simulink model "mpc_simulation_regulation"  (R2022a)
settings: Solver=VariableStepAuto  StartTime=0.0  StopTime=10  RelTol=1e-3
InitFcn:
  | mpc_example_regulation
values from neighbouring files (symbols this model uses):
  absolute_encoder_counts_per_revolution = 128    [ELEN90064_Project_Parameters.m]
  C = [0 1 0 0 0]    [DesignProjectP2.m]    (also in DesignProjectP3.m = [1 0 0 0 0; DesignProject_OffsetP3.m = [1 0 0 0 0; mpc_example_regulation.m = [1 0 0 0 0; mpc_example_tracking.m = [1 0 0 0 0)
  Dp = c2d(Gp, T, 'zoh')    [DesignProject_OffsetP3.m]    (also in mpc_example_regulation.m; mpc_example_tracking.m)
  gyro_sigma_drift = deg2rad(5)    [ELEN90064_Project_Parameters.m]
  init = [theta_m_init; theta_l_init; thetadot_m_init; thetadot_l_init; Ia_init]    [ELEN90064_Project_Parameters.m]
  L_disc = L_disct'    [DesignProject_OffsetP3.m]    (also in mpc_example_regulation.m; mpc_example_tracking.m)
libraries: mpclib x1
settings Model: Creator=pbeuchat  LastModifiedBy=Admin
settings SolverCC: AlgebraicLoopSolver=TrustRegion
settings DebuggingCC: UnconnectedInputMsg=warning  UnconnectedOutputMsg=warning  UnconnectedLineMsg=warning  SFMachineParentedDataDiag=warning
settings RTWCC: DLArmComputeVersion=19.05

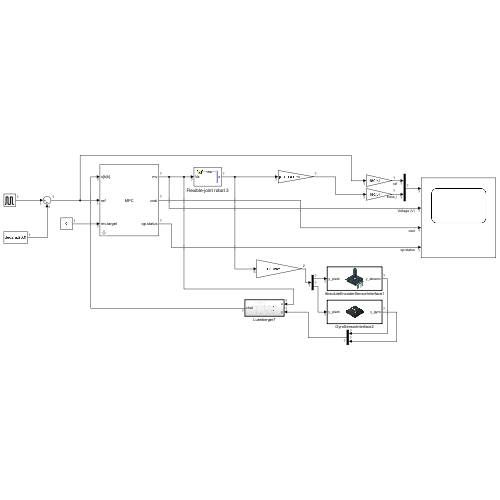
[thumbnail: Simulink's stored preview of the top-level diagram]
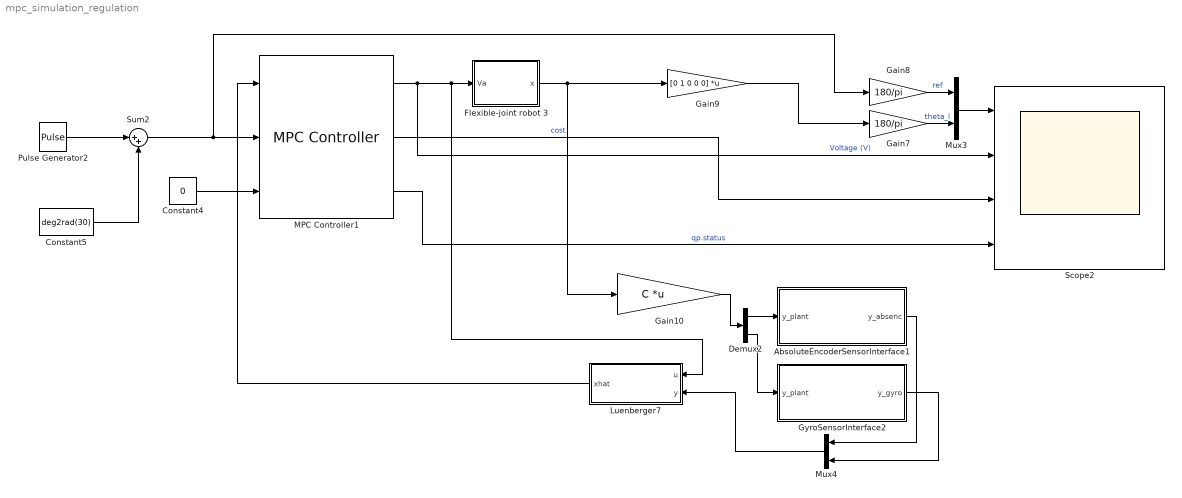
== system mpc_simulation_regulation ==
  AbsoluteEncoderSensorInterface1 : Subsystem  TreatAsAtomicUnit=on
      mask Display: image('$imagefile'); % Use "Edit Image" on toolstrip to change.
  Constant4 : Constant  Value=0
  Constant5 : Constant  Value=deg2rad(30)
  Demux2 : Demux  Outputs=2
  Flexible-joint robot 3 : Subsystem
      mask Display: image('$imagefile'); % Use "Edit Image" on toolstrip to change.
  Gain10 : Gain  Gain=C  Multiplication=Matrix(K*u) (u vector)
  Gain7 : Gain  Gain=180/pi
  Gain8 : Gain  Gain=180/pi
  Gain9 : Gain  Gain=[0 1 0 0 0]  Multiplication=Matrix(K*u)
  GyroSensorInterface2 : Subsystem  TreatAsAtomicUnit=on
      mask Display: image('$imagefile'); % Use "Edit Image" on toolstrip to change.
  Luenberger7 : Subsystem  TreatAsAtomicUnit=on
  MPC Controller1 : mpclib/MPC Controller  SCDEnableBlockLinearizationSpecification=on  mpcobj=mpc_obj  x0=mpc_initial_state  is_multiple=0  enable_value=0  return_u0=off  updateMPCinCallerWorkspace=on  md_inport=off  mv_inport=off  uref_inport=on  return_cost=on  return_mvseq=off  return_qpstatus=on  return_xseq=off  return_state=off  return_ovseq=off  state_inport=on  umin_inport=off  umax_inport=off  ymin_inport=off  ymax_inport=off  cc_inport=off  ywt_inport=off  uwt_inport=off  duwt_inport=off  rhoeps_inport=off  pm_inport=off  MaximumP=10  HorizonChoice=FixedHorizon  n_ts=0.02  n_p=20  n_mv=1  n_md=0  n_ud=0  n_mo=13  n_uo=0  BlockDataType=double  SampleTimeInherited=off  switch_inport=off
  Mux3 : Mux  Inputs=2
  Mux4 : Mux  Inputs=2
  Pulse Generator2 : DiscretePulseGenerator  PulseType=Time based  Amplitude=deg2rad(30)  Period=5  PulseWidth=50
  Scope2 : Scope  NumInputPorts=4
  Sum2 : Sum  Inputs=|++
  wires:
  Gain10/1 -> Demux2/1
  AbsoluteEncoderSensorInterface1/1(y_absenc) -> Mux4/1
  Demux2/1 -> AbsoluteEncoderSensorInterface1/1(y_plant)
  Constant5/1 -> Sum2/2
  Demux2/2 -> GyroSensorInterface2/1(y_plant)
  Constant4/1 -> MPC Controller1/3
  Flexible-joint robot 3/1(x) -> Gain9/1, Gain10/1
  Pulse Generator2/1 -> Sum2/1
  Gain9/1 -> Gain7/1
  GyroSensorInterface2/1(y_gyro) -> Mux4/2
  Gain8/1 -> Mux3/1  "ref"
  Mux3/1 -> Scope2/1
  MPC Controller1/3 -> Scope2/4  "qp.status"
  MPC Controller1/1 -> Luenberger7/1(u), Flexible-joint robot 3/1(Va), Scope2/2  "Voltage (V)"
  MPC Controller1/2 -> Scope2/3  "cost"
  Gain7/1 -> Mux3/2  "theta_l"
  Luenberger7/1(xhat) -> MPC Controller1/1
  Sum2/1 -> MPC Controller1/2, Gain8/1
  Mux4/1 -> Luenberger7/2(y)

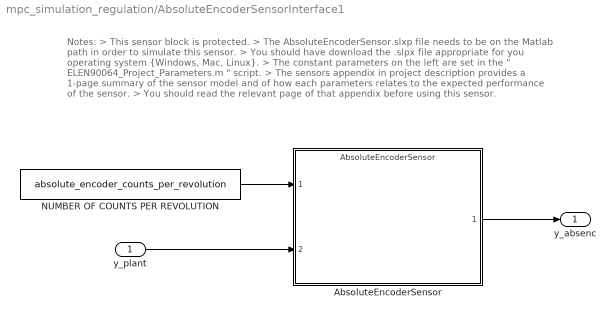
== system mpc_simulation_regulation/AbsoluteEncoderSensorInterface1 ==
  note: Notes:
      | > This sensor block is protected.
      | > The AbsoluteEncoderSensor.slxp file needs to be on the Matlab path in order to simulate this sensor.
      | > You should have download the .slpx file appropriate for you operating system {Windows, Mac, Linux}.
      | > The constant parameters on the left are set in the " ELEN90064_Project_Parameters.m " script.
      | > The sensors appendix in project description provides a 1-page summary of the sensor model and of how each parameters relates to the expected performance of the sensor.
      | > You should read the relevant page of that appendix before using this sensor.
  y_plant : Inport
  AbsoluteEncoderSensor : ModelReference  ModelNameDialog=AbsoluteEncoderSensor.slxp  ModelReferenceVersion=1.16  CopyOfModelProtected=on
  NUMBER OF COUNTS PER REVOLUTION : Constant  Value=absolute_encoder_counts_per_revolution
  y_absenc : Outport
  wires:
  NUMBER OF COUNTS PER REVOLUTION/1 -> AbsoluteEncoderSensor/1
  y_plant/1 -> AbsoluteEncoderSensor/2
  AbsoluteEncoderSensor/1 -> y_absenc/1

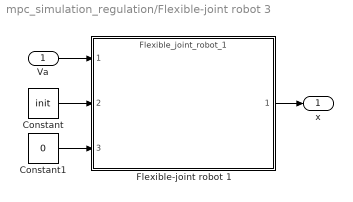
== system mpc_simulation_regulation/Flexible-joint robot 3 ==
  Va : Inport
  Constant : Constant  Value=init
  Constant1 : Constant  Value=0
  Flexible-joint robot 1 : ModelReference  ModelNameDialog=Flexible_joint_robot_1  ModelReferenceVersion=1.65  CopyOfModelProtected=on
  x : Outport
  wires:
  Va/1 -> Flexible-joint robot 1/1
  Flexible-joint robot 1/1 -> x/1
  Constant1/1 -> Flexible-joint robot 1/3
  Constant/1 -> Flexible-joint robot 1/2

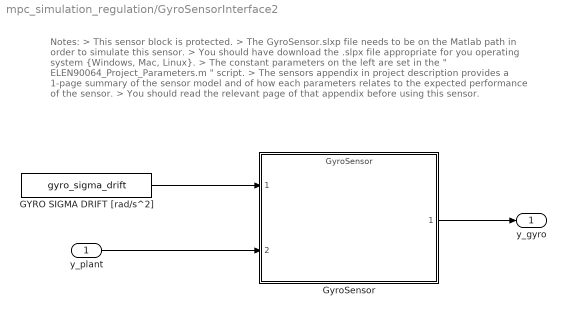
== system mpc_simulation_regulation/GyroSensorInterface2 ==
  note: Notes:
      | > This sensor block is protected.
      | > The GyroSensor.slxp file needs to be on the Matlab path in order to simulate this sensor.
      | > You should have download the .slpx file appropriate for you operating system {Windows, Mac, Linux}.
      | > The constant parameters on the left are set in the " ELEN90064_Project_Parameters.m " script.
      | > The sensors appendix in project description provides a 1-page summary of the sensor model and of how each parameters relates to the expected performance of the sensor.
      | > You should read the relevant page of that appendix before using this sensor.
  y_plant : Inport
  GYRO SIGMA DRIFT [rad/s^2] : Constant  Value=gyro_sigma_drift
  GyroSensor : ModelReference  ModelNameDialog=GyroSensor.slxp  ModelReferenceVersion=1.18  CopyOfModelProtected=on
  y_gyro : Outport
  wires:
  GyroSensor/1 -> y_gyro/1
  y_plant/1 -> GyroSensor/2
  GYRO SIGMA DRIFT [rad/s^2]/1 -> GyroSensor/1

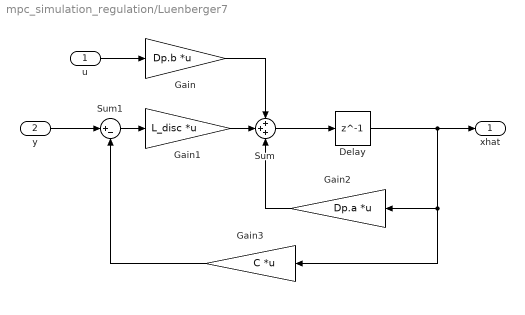
== system mpc_simulation_regulation/Luenberger7 ==
  u : Inport
  y : Inport  Port=2
  Delay : Delay  DelayLength=1
  Gain : Gain  Gain=Dp.b  Multiplication=Matrix(K*u) (u vector)
  Gain1 : Gain  Gain=L_disc  Multiplication=Matrix(K*u) (u vector)
  Gain2 : Gain  Gain=Dp.a  Multiplication=Matrix(K*u) (u vector)
  Gain3 : Gain  Gain=C  Multiplication=Matrix(K*u) (u vector)
  Sum : Sum  Inputs=+++
  Sum1 : Sum  Inputs=|+-
  xhat : Outport
  wires:
  u/1 -> Gain/1
  Gain/1 -> Sum/1
  y/1 -> Sum1/1
  Sum1/1 -> Gain1/1
  Gain1/1 -> Sum/2
  Sum/1 -> Delay/1
  Delay/1 -> Gain3/1, Gain2/1, xhat/1
  Gain2/1 -> Sum/3
  Gain3/1 -> Sum1/2
